simulink model "switch_case_3"  (R2022b)
settings: Solver=VariableStepAuto  StartTime=0.0  StopTime=10.0  RelTol=1e-3
settings Model: Creator=yasso  LastModifiedBy=yasso
settings DebuggingCC: UnconnectedInputMsg=warning  UnconnectedOutputMsg=warning  UnconnectedLineMsg=warning
settings ModelReferenceCC: EnableRefExpFcnMdlSchedulingChecks=on
settings RTWCC: DLArmComputeVersion=19.05

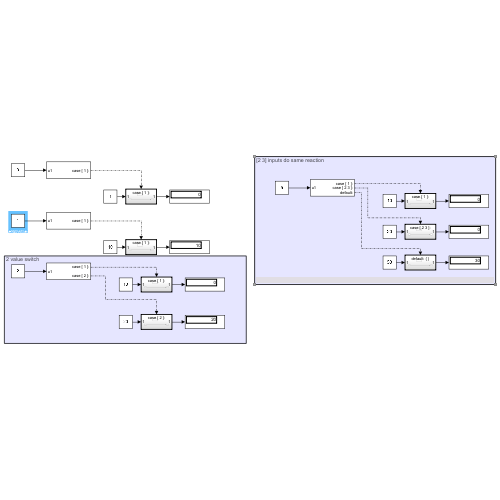
[thumbnail: Simulink's stored preview of the top-level diagram]
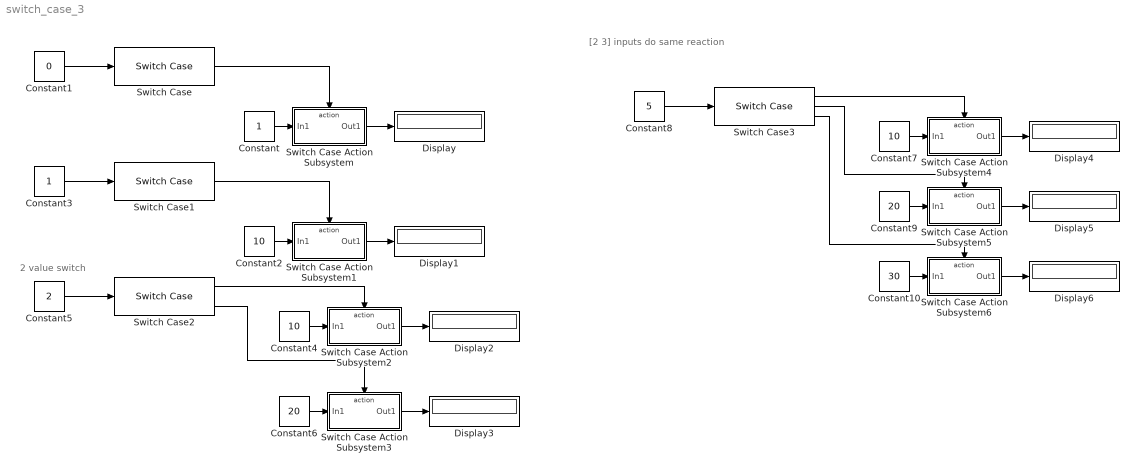
== system switch_case_3 ==
  note: [2 3] inputs do same reaction
  note: 2 value switch
  Constant : Constant
  Constant1 : Constant  Value=0
  Constant10 : Constant  Value=30
  Constant2 : Constant  Value=10
  Constant3 : Constant
  Constant4 : Constant  Value=10
  Constant5 : Constant  Value=2
  Constant6 : Constant  Value=20
  Constant7 : Constant  Value=10
  Constant8 : Constant  Value=5
  Constant9 : Constant  Value=20
  Display{,1..6} (7 alike) : Display
  Switch Case : SwitchCase  ShowDefaultCase=off
  Switch Case Action Subsystem : Subsystem  TreatAsAtomicUnit=on
  Switch Case Action Subsystem1 : Subsystem  TreatAsAtomicUnit=on
  Switch Case Action Subsystem2 : Subsystem  TreatAsAtomicUnit=on
  Switch Case Action Subsystem3 : Subsystem  TreatAsAtomicUnit=on
  Switch Case Action Subsystem4 : Subsystem  TreatAsAtomicUnit=on
  Switch Case Action Subsystem5 : Subsystem  TreatAsAtomicUnit=on
  Switch Case Action Subsystem6 : Subsystem  TreatAsAtomicUnit=on
  Switch Case1 : SwitchCase  ShowDefaultCase=off
  Switch Case2 : SwitchCase  CaseConditions={1,2}  ShowDefaultCase=off
  Switch Case3 : SwitchCase  CaseConditions={1,[2 3]}
  wires:
  Switch Case/1 -> Switch Case Action Subsystem/Action
  Constant/1 -> Switch Case Action Subsystem/1(In1)
  Constant1/1 -> Switch Case/1
  Switch Case Action Subsystem/1(Out1) -> Display/1
  Switch Case1/1 -> Switch Case Action Subsystem1/Action
  Constant2/1 -> Switch Case Action Subsystem1/1(In1)
  Switch Case Action Subsystem1/1(Out1) -> Display1/1
  Constant3/1 -> Switch Case1/1
  Constant5/1 -> Switch Case2/1
  Switch Case Action Subsystem2/1(Out1) -> Display2/1
  Constant4/1 -> Switch Case Action Subsystem2/1(In1)
  Switch Case2/1 -> Switch Case Action Subsystem2/Action
  Constant6/1 -> Switch Case Action Subsystem3/1(In1)
  Switch Case2/2 -> Switch Case Action Subsystem3/Action
  Switch Case Action Subsystem3/1(Out1) -> Display3/1
  Constant8/1 -> Switch Case3/1
  Switch Case3/1 -> Switch Case Action Subsystem4/Action
  Switch Case Action Subsystem4/1(Out1) -> Display4/1
  Switch Case3/2 -> Switch Case Action Subsystem5/Action
  Switch Case Action Subsystem5/1(Out1) -> Display5/1
  Constant7/1 -> Switch Case Action Subsystem4/1(In1)
  Constant9/1 -> Switch Case Action Subsystem5/1(In1)
  Constant10/1 -> Switch Case Action Subsystem6/1(In1)
  Switch Case Action Subsystem6/1(Out1) -> Display6/1
  Switch Case3/3 -> Switch Case Action Subsystem6/Action

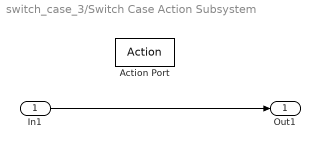
== system switch_case_3/Switch Case Action Subsystem ==
  In1 : Inport
  Action Port : ActionPort  ActionPortLabel=case [ 1 ]:
  Out1 : Outport
  wires:
  In1/1 -> Out1/1

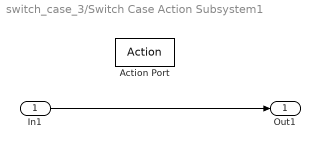
== system switch_case_3/Switch Case Action Subsystem1 ==
  In1 : Inport
  Action Port : ActionPort  ActionPortLabel=case [ 1 ]:
  Out1 : Outport
  wires:
  In1/1 -> Out1/1

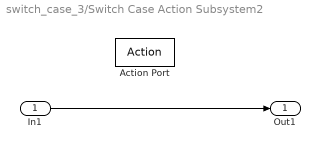
== system switch_case_3/Switch Case Action Subsystem2 ==
  In1 : Inport
  Action Port : ActionPort  ActionPortLabel=case [ 1 ]:
  Out1 : Outport
  wires:
  In1/1 -> Out1/1

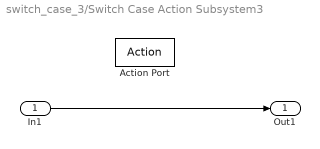
== system switch_case_3/Switch Case Action Subsystem3 ==
  In1 : Inport
  Action Port : ActionPort  ActionPortLabel=case [ 2 ]:
  Out1 : Outport
  wires:
  In1/1 -> Out1/1

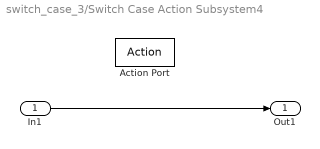
== system switch_case_3/Switch Case Action Subsystem4 ==
  In1 : Inport
  Action Port : ActionPort  ActionPortLabel=case [ 1 ]:
  Out1 : Outport
  wires:
  In1/1 -> Out1/1

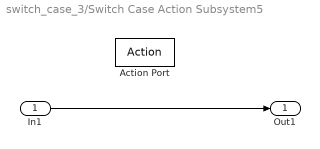
== system switch_case_3/Switch Case Action Subsystem5 ==
  In1 : Inport
  Action Port : ActionPort  ActionPortLabel=case [ 2 3 ]:
  Out1 : Outport
  wires:
  In1/1 -> Out1/1

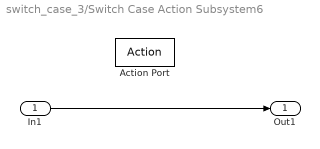
== system switch_case_3/Switch Case Action Subsystem6 ==
  In1 : Inport
  Action Port : ActionPort  ActionPortLabel=default:
  Out1 : Outport
  wires:
  In1/1 -> Out1/1
